simulink model "Hysteresis_Experiment_SimScape_NEURON"  (R2018b)
settings: Solver=VariableStepAuto  StartTime=0.0  StopTime=10.0  RelTol=1e-3
libraries: fl_lib x19, nesl_utility x4, elec_lib x2, simulink x1
settings Model: Creator=dsentc  LastModifiedBy=poker
settings DebuggingCC: LibraryContextMissingDiagnostic=none
settings SFSimCC: SimUseLocalCustomCode=off
settings RTWCC: RTWUseLocalCustomCode=off

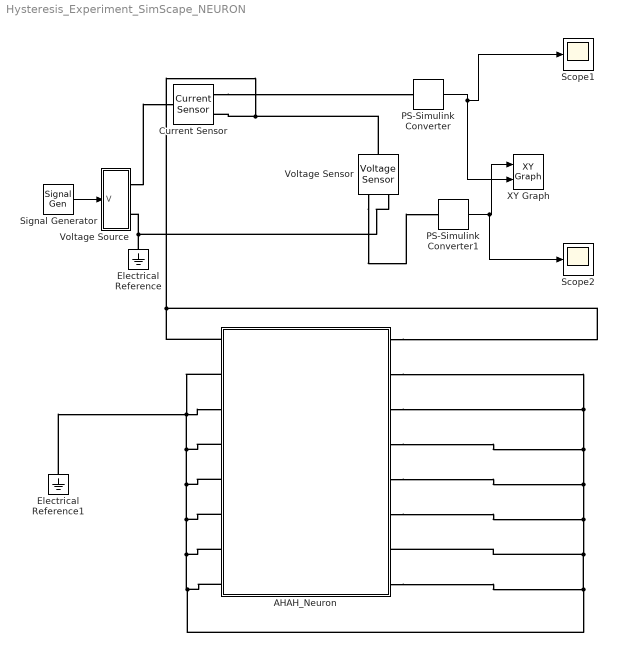
== system Hysteresis_Experiment_SimScape_NEURON ==
  AHAH_Neuron : Subsystem
  Current Sensor : fl_lib/Electrical/Electrical Sensors/Current Sensor
  Electrical Reference : fl_lib/Electrical/Electrical Elements/Electrical Reference
  Electrical Reference1 : fl_lib/Electrical/Electrical Elements/Electrical Reference
  PS-Simulink Converter : nesl_utility/PS-Simulink Converter  PhysicalDomain=network_engine_domain  SubClassName=ps_output  LeftPortType=input  RightPortType=output  PseudoPeriodic=off  Frequencies=[]  Unit=1  AffineConversion=off
  PS-Simulink Converter1 : nesl_utility/PS-Simulink Converter  PhysicalDomain=network_engine_domain  SubClassName=ps_output  LeftPortType=input  RightPortType=output  PseudoPeriodic=off  Frequencies=[]  Unit=1  AffineConversion=off
  Scope1 : Scope
  Scope2 : Scope
  Signal Generator : SignalGenerator  Amplitude=2  Units=rad/sec
  Voltage Source : Subsystem
  Voltage Sensor : fl_lib/Electrical/Electrical Sensors/Voltage Sensor
  XY Graph : simulink/Sinks/XY Graph  xmin=-10  xmax=10  ymin=-10  ymax=10  st=-1
  wires:
  Signal Generator/1 -> Voltage Source/1(V)
  PS-Simulink Converter1/1 -> Scope2/1, XY Graph/1
  PS-Simulink Converter/1 -> Scope1/1, XY Graph/2
  connections:
  Electrical Reference/LConn1 -- Voltage Sensor/RConn2 -- Voltage Source/RConn2
  Voltage Source/RConn1 -- Current Sensor/LConn1
  Voltage Sensor/LConn1 -- AHAH_Neuron/LConn1 -- AHAH_Neuron/RConn1 -- Current Sensor/RConn2
  Current Sensor/RConn1 -- PS-Simulink Converter/LConn1
  Voltage Sensor/RConn1 -- PS-Simulink Converter1/LConn1
  Electrical Reference1/LConn1 -- AHAH_Neuron/LConn3 -- AHAH_Neuron/LConn2 -- AHAH_Neuron/LConn6 -- AHAH_Neuron/RConn7 -- AHAH_Neuron/RConn3 -- AHAH_Neuron/RConn2 -- AHAH_Neuron/RConn4 -- AHAH_Neuron/RConn5 -- AHAH_Neuron/RConn6 -- AHAH_Neuron/RConn8 -- AHAH_Neuron/LConn8 -- AHAH_Neuron/LConn7 -- AHAH_Neuron/LConn5 -- AHAH_Neuron/LConn4

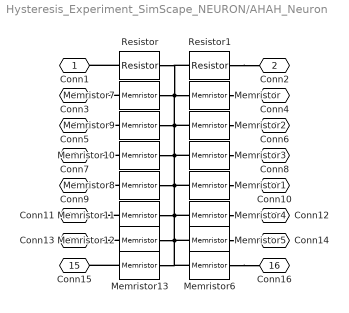
== system Hysteresis_Experiment_SimScape_NEURON/AHAH_Neuron ==
  Memristor{,1..13} (14 alike) : fl_lib/Electrical/Electrical Elements/Memristor  Ra=1 Ohm  Rb=1e2 Ohm  Q0=1e-2 C  x0=0  pwindow=2  i_specify=off  i_priority=None  i=0 A  i_nominal_specify=off  i_nominal_unit=A  i_nominal_value=1  v_specify=off  v_priority=None  v=0 V  v_nominal_specify=off  v_nominal_unit=V  v_nominal_value=1
      settings: SourceProductName=Simscape  SourceProductBaseCode=SS
  Resistor : elec_lib/Passive Devices/Resistor  R=0.0000001 Ohm  R_tol=5  enable_R_tol=0  tol_distribution=1  nSigma=4  enable_operating_limits=0  operating_limit_action=2  max_working_voltage=100 V  power_rating=1 W  enable_faults=0  fault_action=1  R_faulted=inf Ohm  enable_temporal_fault=0  t_fault=1 s  enable_behavioral_fault=0  max_permissible_current=1 A  t_fail_on_current=1 s  noise_mode=0  sample_time=1e-3 s  repeatability=1  auto_seed=641212872  user_seed=0  Tdevice=25 degC  alpha=3.93e-3 1/K  Tmeas=25 degC  thermal_mass=100 J/K  power_derating_T1=70 degC  power_derating_T2=155 degC  operating_temperature_range_vec=[-50, 150] degC  temperature_specify=off  temperature_priority=High  temperature=298.15 K  temperature_nominal_specify=off  temperature_nominal_unit=K  temperature_nominal_value=1
  Resistor1 : elec_lib/Passive Devices/Resistor  R=0.0000001 Ohm  R_tol=5  enable_R_tol=0  tol_distribution=1  nSigma=4  enable_operating_limits=0  operating_limit_action=2  max_working_voltage=100 V  power_rating=1 W  enable_faults=0  fault_action=1  R_faulted=inf Ohm  enable_temporal_fault=0  t_fault=1 s  enable_behavioral_fault=0  max_permissible_current=1 A  t_fail_on_current=1 s  noise_mode=0  sample_time=1e-3 s  repeatability=1  auto_seed=1105989530  user_seed=0  Tdevice=25 degC  alpha=3.93e-3 1/K  Tmeas=25 degC  thermal_mass=100 J/K  power_derating_T1=70 degC  power_derating_T2=155 degC  operating_temperature_range_vec=[-50, 150] degC  temperature_specify=off  temperature_priority=High  temperature=298.15 K  temperature_nominal_specify=off  temperature_nominal_unit=K  temperature_nominal_value=1
  Conn1 : PMIOPort  Side=Left
  Conn2 : PMIOPort  Port=2  Side=Right
  Conn3 : PMIOPort  Port=3  Side=Left
  Conn4 : PMIOPort  Port=4  Side=Right
  Conn5 : PMIOPort  Port=5  Side=Left
  Conn6 : PMIOPort  Port=6  Side=Right
  Conn7 : PMIOPort  Port=7  Side=Left
  Conn8 : PMIOPort  Port=8  Side=Right
  Conn9 : PMIOPort  Port=9  Side=Left
  Conn10 : PMIOPort  Port=10  Side=Right
  Conn11 : PMIOPort  Port=11  Side=Left
  Conn12 : PMIOPort  Port=12  Side=Right
  Conn13 : PMIOPort  Port=13  Side=Left
  Conn14 : PMIOPort  Port=14  Side=Right
  Conn15 : PMIOPort  Port=15  Side=Left
  Conn16 : PMIOPort  Port=16  Side=Right
  connections:
  Memristor10/RConn1 -- Conn7/RConn1
  Memristor7/LConn1 -- Resistor1/LConn1 -- Resistor/RConn1 -- Memristor3/LConn1 -- Memristor1/LConn1 -- Memristor4/LConn1 -- Memristor6/LConn1 -- Memristor13/LConn1 -- Memristor5/LConn1 -- Memristor12/LConn1 -- Memristor11/LConn1 -- Memristor8/LConn1 -- Memristor10/LConn1 -- Memristor2/LConn1 -- Memristor9/LConn1 -- Memristor/LConn1
  Memristor5/RConn1 -- Conn14/RConn1
  Memristor11/RConn1 -- Conn11/RConn1
  Resistor1/RConn1 -- Conn2/RConn1
  Memristor3/RConn1 -- Conn8/RConn1
  Memristor13/RConn1 -- Conn15/RConn1
  Memristor6/RConn1 -- Conn16/RConn1
  Memristor4/RConn1 -- Conn12/RConn1
  Resistor/LConn1 -- Conn1/RConn1
  Memristor2/RConn1 -- Conn6/RConn1
  Memristor1/RConn1 -- Conn10/RConn1
  Memristor7/RConn1 -- Conn3/RConn1
  Memristor9/RConn1 -- Conn5/RConn1
  Memristor8/RConn1 -- Conn9/RConn1
  Memristor12/RConn1 -- Conn13/RConn1
  Memristor/RConn1 -- Conn4/RConn1

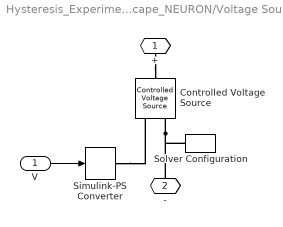
== system Hysteresis_Experiment_SimScape_NEURON/Voltage Source ==
  V : Inport
  Controlled Voltage Source : fl_lib/Electrical/Electrical Sources/Controlled Voltage Source
  Simulink-PS Converter : nesl_utility/Simulink-PS Converter  PhysicalDomain=network_engine_domain  SubClassName=ps_input  LeftPortType=input  RightPortType=output  PseudoPeriodic=off  Frequencies=[]  NoiseDistribution=none  NoiseParameters=[]  Unit=1  AffineConversion=off  FilteringAndDerivatives=zero  SimscapeFilterOrder=1  InputFilterTimeConstant=.001  UdotUserProvided=0
  Solver Configuration : nesl_utility/Solver Configuration  PhysicalDomain=network_engine_domain  SubClassName=solver  LeftPortType=input  RightPortType=generic  Tones=[]  Harmonics=[]  SimulateNoise=off  Profile=off  UseLocalSampling=off  EnableSwitchedLinearOptims=on  FrequencyDomain=off  UseCCode=off  RelTol=0.001  AbsTol=1e-06  MinStep=1e-09  ToWorkspace=off  RevertToSquareIcSolve=off  NumHomotopyIterations=100  PhasorMode=off  PhasorModeNumHarmonics=1  DoDC=off  ResidualTolerance=1e-9  UseLocalSolver=off  LocalSolverChoice=NE_BACKWARD_EULER_ADVANCER  LocalSolverSampleTime=.001  DoFixedCost=off  MaxNonlinIter=3  MaxModeIter=2  LinearAlgebra=Sparse  EquationFormulation=NE_TIME_EF  DelaysMemoryBudget=1024  AutomaticFiltering=on  FilteringTimeConstant=0.001  PartitionStorageMethod=AS_NEEDED  PartitionMemoryBudget=1024
  + : PMIOPort  Side=Right
  - : PMIOPort  Port=2  Side=Right
  wires:
  V/1 -> Simulink-PS Converter/1
  connections:
  Simulink-PS Converter/RConn1 -- Controlled Voltage Source/RConn1
  Controlled Voltage Source/RConn2 -- -/RConn1 -- Solver Configuration/RConn1
  +/RConn1 -- Controlled Voltage Source/LConn1
